simulink model "Simulation"  (R2018b)
settings: Solver=VariableStepAuto  StartTime=0.0  StopTime=tmax  RelTol=1e-3
undefined symbols (not defined in the file): Kd, Ki, Kp, V
libraries: simulink_extras x3
settings Model: Creator=fieri  LastModifiedBy=fieri
settings SolverCC: MaxConsecutiveMinStep=10  ZeroCrossAlgorithm=Adaptive

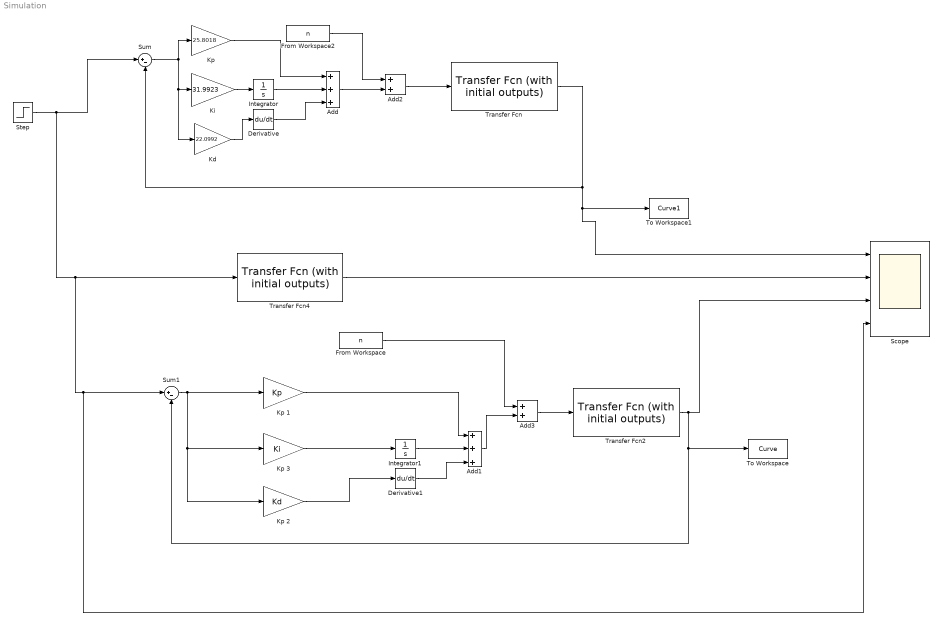
== system Simulation ==
  Add : Sum  Inputs=+++
  Add1 : Sum  Inputs=+++
  Add2 : Sum
  Add3 : Sum
  Derivative : Derivative
  Derivative1 : Derivative
  From Workspace : FromWorkspace  VariableName=n  SampleTime=0
  From Workspace2 : FromWorkspace  VariableName=n  SampleTime=0
  Integrator : Integrator
  Integrator1 : Integrator
  Kd : Gain  Gain=22.0992
  Ki : Gain  Gain=31.9923
  "Kp " : Gain  Gain=25.8018
  Kp 1 : Gain  Gain=Kp
  Kp 2 : Gain  Gain=Kd
  Kp 3 : Gain  Gain=Ki
  Scope : Scope  NumInputPorts=4
  Step : Step  Before=V  After=V  SampleTime=0
  Sum : Sum  Inputs=|+-
  Sum1 : Sum  Inputs=|+-
  To Workspace : ToWorkspace  VariableName=Curve  SampleTime=1
  To Workspace1 : ToWorkspace  VariableName=Curve1  SampleTime=1
  Transfer Fcn : simulink_extras/Additional Linear/Transfer Fcn (with initial outputs)  N=[0.2608]  D="[1  1.281 0.2615]"  Y0=0  U0=0
  Transfer Fcn2 : simulink_extras/Additional Linear/Transfer Fcn (with initial outputs)  N=[0.2608]  D="[1  1.281 0.2615]"  Y0=0  U0=0
  Transfer Fcn4 : simulink_extras/Additional Linear/Transfer Fcn (with initial outputs)  N=[0.2608]  D="[1  1.281 0.2615]"  Y0=0  U0=0
  wires:
  Kd/1 -> Derivative/1
  Derivative/1 -> Add/3
  Ki/1 -> Integrator/1
  Integrator/1 -> Add/2
  "Kp "/1 -> Add/1
  Sum/1 -> Kd/1, Ki/1, "Kp "/1
  Derivative1/1 -> Add1/3
  Integrator1/1 -> Add1/2
  Sum1/1 -> Kp 2/1, Kp 3/1, Kp 1/1
  Kp 3/1 -> Integrator1/1
  Kp 2/1 -> Derivative1/1
  Kp 1/1 -> Add1/1
  Add1/1 -> Add3/2
  Add3/1 -> Transfer Fcn2/1
  Add/1 -> Add2/2
  Add2/1 -> Transfer Fcn/1
  From Workspace2/1 -> Add2/1
  From Workspace/1 -> Add3/1
  Transfer Fcn/1 -> To Workspace1/1, Scope/1, Sum/2
  Transfer Fcn4/1 -> Scope/2
  Transfer Fcn2/1 -> Scope/3, Sum1/2, To Workspace/1
  Step/1 -> Scope/4, Sum1/1, Transfer Fcn4/1, Sum/1
